simulink model "ThyristorRectifier"  (R2023b)
settings: Solver=FixedStepAuto  StartTime=0.0  StopTime=0.08333  FixedStep=Ts  MaxStep=1e-4  RelTol=1e-3  EnableMultiTasking=on
PreLoadFcn:
  | Ts = 1e-5;
libraries: nesl_utility x10, ee_lib x7, fl_lib x3, eeThyristorSixPulseGenerator x1, eeSinusoidalMeasurement x1
CloseFcn:
  | clear simlog_ThyristorRectifier
  | clear logsout_ThyristorRectifier
Description:
  | Thyristor-Based Rectifier
settings Model: Creator=The MathWorks, Inc.  LastModifiedBy=abdulkadir
settings SolverCC: AlgebraicLoopSolver=TrustRegion
settings DataIOCC: MaxDataPoints=15000  SaveFormat=Array  SaveOutput=off  SaveTime=off  ReturnWorkspaceOutputs=off  SignalLoggingName=logsout_ThyristorRectifier
settings OptimizationCC: ReuseModelBlockBuffer=off  LifeSpan=inf
settings DebuggingCC: UnderspecifiedInitializationDetection=Classic  MergeDetectMultiDrivingBlocksExec=none  SolverPrmCheckMsg=warning  UnconnectedInputMsg=warning  UnconnectedOutputMsg=warning  UnconnectedLineMsg=warning  SFUnexpectedBacktrackingDiag=warning  SFNoUnconditionalDefaultTransitionDiag=warning  SFExecutionAtInitializationDiag=none  ArithmeticOperatorsInVariantConditions=warning
settings HardwareCC: ProdBitPerPointer=32  ProdBitPerSizeT=32  ProdBitPerPtrDiffT=32  ProdLargestAtomicFloat=None  ProdIntDivRoundTo=Undefined  ProdEndianess=Unspecified  ProdWordSize=32  ProdHWDeviceType=32-bit Generic
settings ModelReferenceCC: EnableRefExpFcnMdlSchedulingChecks=on  PropagateSignalLabelsOutOfModel=off
settings SFSimCC: SimUseLocalCustomCode=off  CustomCodeUndefinedFunction=UseInterfaceOnly
settings RTWCC: RTWUseLocalCustomCode=off  DLArmComputeVersion=19.05
settings CodeAppCC: StateflowObjectComments=on
settings GRTTargetCC: TargetLangStandard=C89/C90 (ANSI)
settings ConfigComp: CovMetricSettings=dw  CovSaveCumulativeToWorkspaceVar=on  CovSaveSingleToWorkspaceVar=on  CovExternalEMLEnable=off
settings SimscapeCC: SimscapeLogType=all  SimscapeLogSimulationStatistics=on  SimscapeLogName=simlog_ThyristorRectifier  SimscapeLogDataHistory=15000

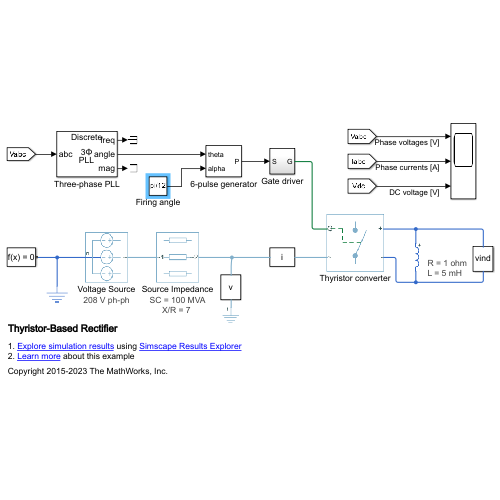
[thumbnail: Simulink's stored preview of the top-level diagram]
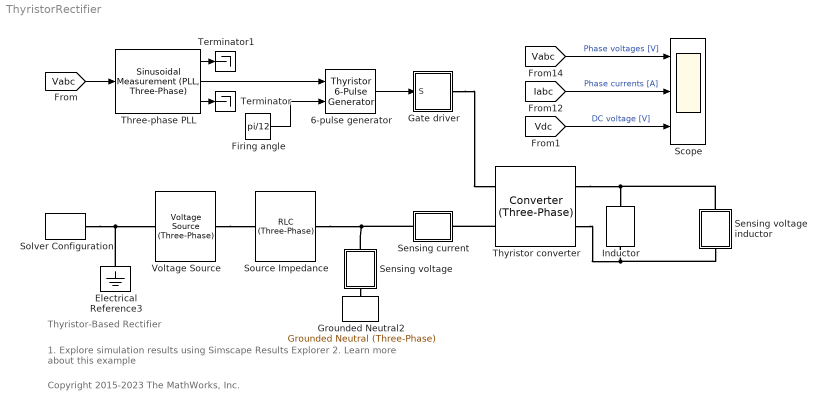
== system ThyristorRectifier ==
  note: 1. Explore simulation results using Simscape Results Explorer
      | 2. Learn more about this example
  note: Thyristor-Based Rectifier
  note: Copyright 2015-2023 The MathWorks, Inc.
  6-pulse generator : eeThyristorSixPulseGenerator/Thyristor 6-Pulse Generator  Ord=Sequential device order  Pw=5*pi/6  Ts=1e-5
  Electrical Reference3 : fl_lib/Electrical/Electrical Elements/Electrical Reference
  Firing angle : Constant  Value=pi/12  SampleTime=Ts
  Gate driver : Subsystem
  Grounded Neutral2 : ee_lib/Connectors & References/Grounded Neutral (Three-Phase)
  Inductor : fl_lib/Electrical/Electrical Elements/Inductor  l=5e-3 H  r=1 Ohm  g=1e-9 1/Ohm  i_specify=off  i_priority=High  i=0 A  i_nominal_specify=off  i_nominal_unit=A  i_nominal_value=1  v_specify=off  v_priority=High  v=0 V  v_nominal_specify=off  v_nominal_unit=V  v_nominal_value=1  i_L_specify=on  i_L_priority=High  i_L=0 A  i_L_nominal_specify=off  i_L_nominal_unit=A  i_L_nominal_value=1
      settings: AttributesFormatString=|
      | R = 1 ohm
      | L = 5 mH
  Scope : Scope  NumInputPorts=3
  Sensing current : Subsystem
      mask Display: disp('i')
  Sensing voltage : Subsystem
      mask Display: disp('v')
  "Sensing voltage inductor " : Subsystem
      mask Display: disp('vind')
  Solver Configuration : nesl_utility/Solver Configuration  PhysicalDomain=network_engine_domain  SubClassName=solver  LeftPortType=input  RightPortType=generic  Tones=[]  Harmonics=[]  SimulateNoise=off  Profile=off  UseLocalSampling=off  EnableSwitchedLinearOptims=on  FrequencyDomain=off  UseCCode=off  RelTol=0.001  AbsTol=1e-06  MinStep=1e-09  ToWorkspace=off  RevertToSquareIcSolve=off  NumHomotopyIterations=100  PhasorMode=off  PhasorModeNumHarmonics=1  ConsistencySolver=NEWTON_FTOL  IndexReductionMethod=DerivativeReplacement  DoDC=off  ResidualTolerance=1e-9  ConsistencyTolSource=GLOBAL  ConsistencyAbsTol=0.001  ConsistencyRelTol=0.001  ConsistencyTolFactor=0.001  UseLocalSolver=on  LocalSolverChoice=NE_BACKWARD_EULER_ADVANCER  ResolveIndetEquations=on  FunctionEvalNumThread=1  LocalSolverSampleTime=Ts  DoFixedCost=off  MaxNonlinIter=3  MaxModeIter=2  ComputeImpulses=off  ImpulseIterations=2  LinearAlgebra=auto  LinearAlgebraNumThread=0  EquationFormulation=NE_TIME_EF  DelaysMemoryBudget=1024  AutomaticFiltering=on  FilteringTimeConstant=0.001  PartitionStorageMethod=AS_NEEDED  PartitionMemoryBudget=1024  PartitionMethod=FAST  MultibodyUseLocalSolver=off  MultibodyLocalSolverChoice=ODE1  MultibodyLocalSolverSampleTime=0.001
  Source Impedance : ee_lib/Passive/RLC Assemblies/RLC (Three-Phase)  component_structure=4  R=(120*sqrt(3))^2/(100e6*60) / 7 Ohm  L=(120*sqrt(3))^2/(100e6*2*pi*60) H  C=1e-6 F  R_parasitic=1e-6 Ohm  G_parasitic=1e-6 1/Ohm  IL_specify=on  IL_priority=High  IL=[ 0 0 0 ] A  IL_nominal_specify=off  IL_nominal_unit=A  IL_nominal_value=1  VC_specify=on  VC_priority=High  VC=[ 0 0 0 ] V  VC_nominal_specify=off  VC_nominal_unit=V  VC_nominal_value=1
      settings: InternalSimscapePortConfiguration="{\"Bottom\":[],\"Left\":[{\"id\":\"N1\",\"label\":\"~1\",\"type\":\"foundation.electrical.three_phase\"}],\"Right\":[{\"id\":\"N2\",\"label\":\"~2\",\"type\":\"foundation.electrical.three_phase\"}],\"Top\":[]}"
      settings: AttributesFormatString=|
      | SC = 100 MVA
      | X/R = 7
  Terminator : Terminator
  Terminator1 : Terminator
  Three-phase PLL : eeSinusoidalMeasurement/Sinusoidal Measurement (PLL, Three-Phase)  Kp_LF=45  Ki_LF=1250  F0=60  Theta0=0  Ts=Ts
  Thyristor converter : ee_lib/Semiconductors & Converters/Converters/Converter (Three-Phase)  port_option=ee.enum.threePhasePort.composite  device_type=5  K=0  Vf=0.8 V  Ron=0.001 Ohm  Rds=0.001 Ohm  Goff=1e-5 1/Ohm  Vgt=.5 V  Vgt_off=-1 V  Ih=1 A  Vth=6 V  diode_param=1  diode_Vf=0.8 V  diode_Ron=0.001 Ohm  diode_Goff=1e-5 1/Ohm  diode_C=50 nF  diode_iRM=-235 A  diode_iF=300 A  diode_idot=-50 A/us  diode_trr_param=1  diode_trr_factor=3  diode_trr=15 us  diode_Qrr=1.5e+3 s*uA  snubber_type=ee.enum.converters.snubber.exclude  Cs=1e-7 F  Rs=0.1 Ohm
  Voltage Source : ee_lib/Sources/Voltage Source (Three-Phase)  vline_rms=120*sqrt(3) V  shift=0 deg  freq=50 Hz  impedance_option=0  SShortCircuit=1e6 V*A  XR=15  R=0.01 Ohm  L=3.97e-4 H  harmonic_option=0  harmonic_orders=[5, 7, 11, 13]  harmonic_ratios=[0.1, 0.1, 0.1, 0.1]  G_parasitic=0 1/Ohm  I_specify=off  I_priority=None  I=[ 0 0 0 ] A  I_nominal_specify=off  I_nominal_unit=A  I_nominal_value=1
      settings: AttributesFormatString=208 V ph-ph
  wires:
  [Vabc] -> Scope/1  "Phase voltages [V]"
  [Iabc] -> Scope/2  "Phase currents [A]"
  [Vdc] -> Scope/3  "DC voltage [V]"
  Three-phase PLL/2 -> 6-pulse generator/1
  [Vabc] -> Three-phase PLL/1
  6-pulse generator/1 -> Gate driver/1(S)
  Firing angle/1 -> 6-pulse generator/2
  Three-phase PLL/3 -> Terminator/1
  Three-phase PLL/1 -> Terminator1/1
  connections:
  Electrical Reference3/LConn1 -- Voltage Source/LConn1 -- Solver Configuration/RConn1
  Source Impedance/RConn1 -- Sensing current/LConn1 -- Sensing voltage/LConn1
  Voltage Source/RConn1 -- Source Impedance/LConn1
  Thyristor converter/LConn2 -- Sensing current/RConn1
  Gate driver/RConn1 -- Thyristor converter/LConn1
  Sensing voltage/RConn1 -- Grounded Neutral2/LConn1
  Thyristor converter/RConn2 -- "Sensing voltage inductor "/LConn1 -- Inductor/RConn1
  Thyristor converter/RConn1 -- "Sensing voltage inductor "/RConn1 -- Inductor/LConn1

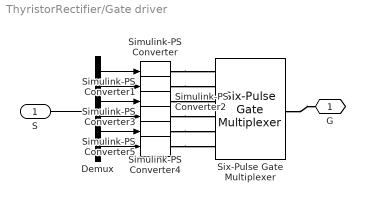
== system ThyristorRectifier/Gate driver ==
  S : Inport
  Demux : Demux  Outputs=6
  Simulink-PS Converter{,1..5} (6 alike) : nesl_utility/Simulink-PS Converter  PhysicalDomain=network_engine_domain  SubClassName=ps_input  LeftPortType=input  RightPortType=output  PseudoPeriodic=off  Frequencies=[]  NoiseDistribution=none  NoiseParameters=[]  Unit=1  AffineConversion=off  FilteringAndDerivatives=zero  SimscapeFilterOrder=1  InputFilterTimeConstant=0.001  UdotUserProvided=0
  Six-Pulse Gate Multiplexer : ee_lib/Semiconductors & Converters/Converters/Six-Pulse Gate Multiplexer  port_option=ee.enum.controlport.ps
  G : PMIOPort  Side=Right
  wires:
  Demux/1 -> Simulink-PS Converter/1
  Demux/5 -> Simulink-PS Converter4/1
  Demux/2 -> Simulink-PS Converter1/1
  Demux/4 -> Simulink-PS Converter3/1
  S/1 -> Demux/1
  Demux/3 -> Simulink-PS Converter2/1
  Demux/6 -> Simulink-PS Converter5/1
  connections:
  Six-Pulse Gate Multiplexer/RConn1 -- G/RConn1
  Simulink-PS Converter4/RConn1 -- Six-Pulse Gate Multiplexer/LConn5
  Simulink-PS Converter/RConn1 -- Six-Pulse Gate Multiplexer/LConn1
  Simulink-PS Converter3/RConn1 -- Six-Pulse Gate Multiplexer/LConn4
  Simulink-PS Converter2/RConn1 -- Six-Pulse Gate Multiplexer/LConn3
  Simulink-PS Converter1/RConn1 -- Six-Pulse Gate Multiplexer/LConn2
  Simulink-PS Converter5/RConn1 -- Six-Pulse Gate Multiplexer/LConn6

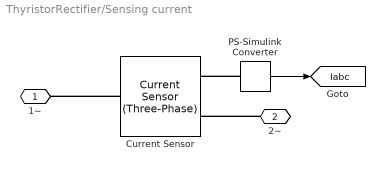
== system ThyristorRectifier/Sensing current ==
  Current Sensor : ee_lib/Sensors & Transducers/Current Sensor (Three-Phase)
  PS-Simulink Converter : nesl_utility/PS-Simulink Converter  PhysicalDomain=network_engine_domain  SubClassName=ps_output  LeftPortType=input  RightPortType=output  PseudoPeriodic=off  Frequencies=[]  VectorFormat=1-D array  Unit=A  AffineConversion=off
  1~ : PMIOPort  Side=Left
  2~ : PMIOPort  Port=2  Side=Right
  tag scope: Iabc=global
  wires:
  PS-Simulink Converter/1 -> [Iabc]
  connections:
  2~/RConn1 -- Current Sensor/RConn2
  PS-Simulink Converter/LConn1 -- Current Sensor/RConn1
  Current Sensor/LConn1 -- 1~/RConn1

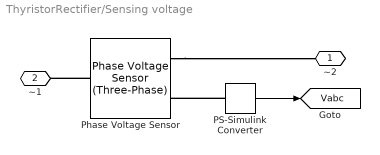
== system ThyristorRectifier/Sensing voltage ==
  PS-Simulink Converter : nesl_utility/PS-Simulink Converter  PhysicalDomain=network_engine_domain  SubClassName=ps_output  LeftPortType=input  RightPortType=output  PseudoPeriodic=off  Frequencies=[]  VectorFormat=1-D array  Unit=V  AffineConversion=off
  Phase Voltage Sensor : ee_lib/Sensors & Transducers/Phase Voltage Sensor (Three-Phase)
  ~2 : PMIOPort  Side=Right
  ~1 : PMIOPort  Port=2  Side=Left
  tag scope: Vabc=global
  wires:
  PS-Simulink Converter/1 -> [Vabc]
  connections:
  Phase Voltage Sensor/LConn1 -- ~1/RConn1
  Phase Voltage Sensor/RConn2 -- ~2/RConn1
  PS-Simulink Converter/LConn1 -- Phase Voltage Sensor/RConn1

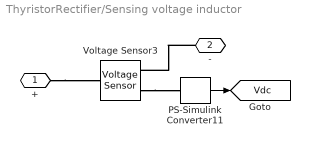
== system ThyristorRectifier/Sensing voltage inductor  ==
  PS-Simulink Converter11 : nesl_utility/PS-Simulink Converter  PhysicalDomain=network_engine_domain  SubClassName=ps_output  LeftPortType=input  RightPortType=output  PseudoPeriodic=off  Frequencies=[]  VectorFormat=1-D array  Unit=1  AffineConversion=off
  Voltage Sensor3 : fl_lib/Electrical/Electrical Sensors/Voltage Sensor
  + : PMIOPort  Side=Left
  - : PMIOPort  Port=2  Side=Right
  tag scope: Vdc=global
  wires:
  PS-Simulink Converter11/1 -> [Vdc]
  connections:
  +/RConn1 -- Voltage Sensor3/LConn1
  Voltage Sensor3/RConn1 -- PS-Simulink Converter11/LConn1
  -/RConn1 -- Voltage Sensor3/RConn2
